simulink model "TorqueVectoring"  (R2021b)
settings: Solver=FixedStepDiscrete  StartTime=0.0  StopTime=10.0  FixedStep=0.001  RelTol=1e-3
model workspace (MAT data in the model file):
  DeadzoneYawrateError = 10
  SteeringDeadzonelimit = 10
values from neighbouring files (symbols this model uses):
  feedforwardgain = 4    [Controllerparameters.m]
  g = 9.81    [Controllerparameters.m]
  Gr = 12    [Controllerparameters.m]
  Ku = 0    [Controllerparameters.m]
  l = 1.53    [Controllerparameters.m]
  LowerYawMoment = -3600    [Controllerparameters.m]
  myy = 2    [Controllerparameters.m]
  Rd = 0.205    [Controllerparameters.m]
  Sgr = 5    [Controllerparameters.m]
  UpperYawMoment = 3600    [Controllerparameters.m]
  wf = 0.6    [Controllerparameters.m]
  wr = 0.6    [Controllerparameters.m]
libraries: simulink x1, mpclib x1
settings Model: Creator=E101180  LastModifiedBy=eiakim
settings OptimizationCC: DefaultParameterBehavior=Inlined  UseDivisionForNetSlopeComputation=on  GainParamInheritBuiltInType=on  UseFloatMulNetSlope=on  InlineInvariantSignals=on  PassReuseOutputArgsAs=Individual arguments  ZeroExternalMemoryAtStartup=off  ZeroInternalMemoryAtStartup=off  NoFixptDivByZeroProtection=on  EfficientFloat2IntCast=on  LifeSpan=1  OptimizeBlockOrder=speed  DifferentSizesBufferReuse=on  EfficientTunableParamExpr=on
settings DebuggingCC: ParameterTunabilityLossMsg=error  UnconnectedInputMsg=none  UnconnectedOutputMsg=none  UnconnectedLineMsg=none
settings HardwareCC: ProdBitPerPointer=32  ProdBitPerSizeT=32  ProdBitPerPtrDiffT=32  ProdLargestAtomicInteger=Long  ProdLargestAtomicFloat=Double  ProdWordSize=32  ProdLongLongMode=on  ProdHWDeviceType=ARM Compatible->ARM Cortex-M
settings ModelReferenceCC: EnableRefExpFcnMdlSchedulingChecks=off
settings SFSimCC: MATLABDynamicMemAlloc=off
settings RTWCC: Description=Embedded Coder  SystemTargetFile=ert.tlc  TemplateMakefile=ert_default_tmf  DLArmComputeVersion=20.02.1
settings CodeAppCC: ForceParamTrailComments=on  IgnoreCustomStorageClasses=off  OperatorAnnotations=on  SimulinkDataObjDesc=on  SFDataObjDesc=on  CustomSymbolStrGlobalVar=rt$N$M  CustomSymbolStrType=$N$M  CustomSymbolStrFcn=$N$M$F  CustomSymbolStrMacro=$N$M  InsertBlockDesc=on
settings ERTTargetCC: TargetLangStandard=C99 (ISO)  GenerateSampleERTMain=on  IncludeMdlTerminateFcn=off  CombineSignalStateStructs=on  SupportAbsoluteTime=off  SupportComplex=off  SupportNonInlinedSFcns=on  InlinedParameterPlacement=NonHierarchical  ERTCustomFileTemplate=example_file_process.tlc  ERTFilePackagingFormat=CompactWithDataFile

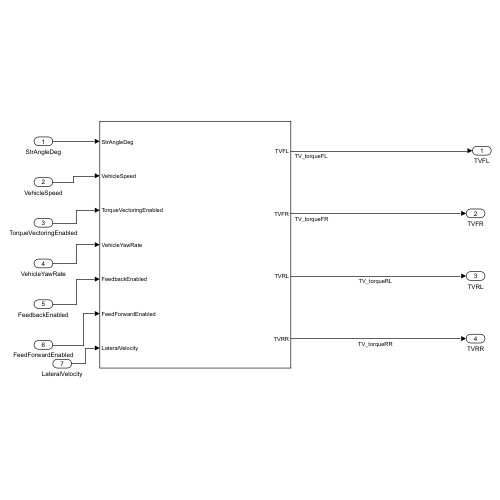
[thumbnail: Simulink's stored preview of the top-level diagram]
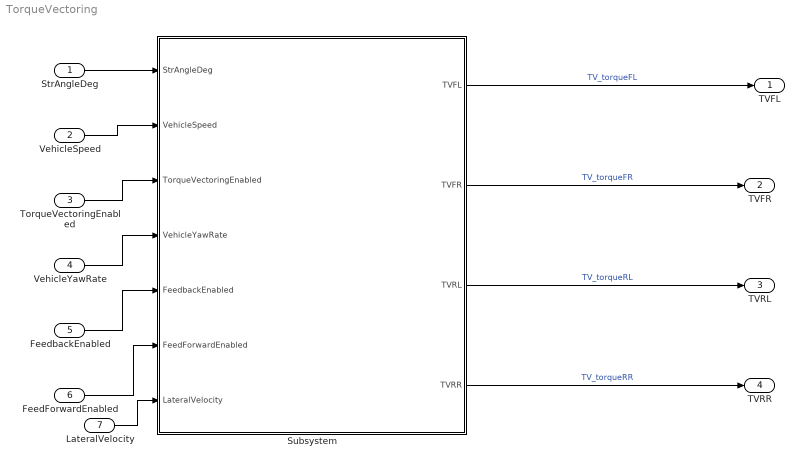
== system TorqueVectoring ==
  StrAngleDeg : Inport
  VehicleSpeed : Inport  Port=2
  TorqueVectoringEnabled : Inport  Port=3
  VehicleYawRate : Inport  Port=4
  FeedbackEnabled : Inport  Port=5
  FeedForwardEnabled : Inport  Port=6
  LateralVelocity : Inport  Port=7
  Subsystem : Subsystem
  TVFL : Outport
  TVFR : Outport  Port=2
  TVRL : Outport  Port=3
  TVRR : Outport  Port=4
  wires:
  Subsystem/3(TVRL) -> TVRL/1  "TV_torqueRL"
  Subsystem/4(TVRR) -> TVRR/1  "TV_torqueRR"
  Subsystem/1(TVFL) -> TVFL/1  "TV_torqueFL"
  StrAngleDeg/1 -> Subsystem/1(StrAngleDeg)
  VehicleSpeed/1 -> Subsystem/2(VehicleSpeed)
  TorqueVectoringEnabled/1 -> Subsystem/3(TorqueVectoringEnabled)
  FeedForwardEnabled/1 -> Subsystem/6(FeedForwardEnabled)
  FeedbackEnabled/1 -> Subsystem/5(FeedbackEnabled)
  VehicleYawRate/1 -> Subsystem/4(VehicleYawRate)
  Subsystem/2(TVFR) -> TVFR/1  "TV_torqueFR"
  LateralVelocity/1 -> Subsystem/7(LateralVelocity)

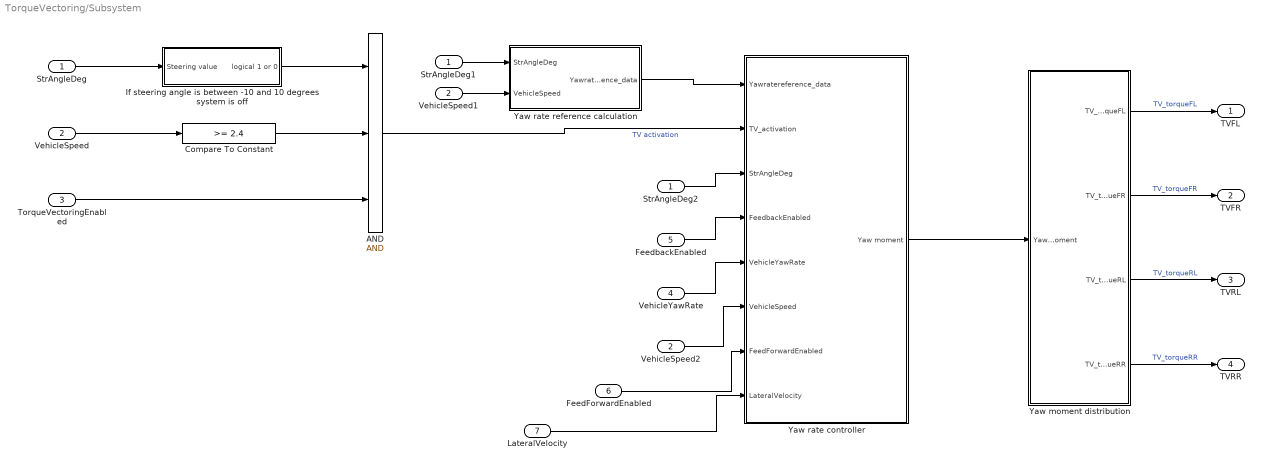
== system TorqueVectoring/Subsystem ==
  StrAngleDeg : Inport
  VehicleSpeed : Inport  Port=2
  TorqueVectoringEnabled : Inport  Port=3
  VehicleYawRate : Inport  Port=4
  FeedbackEnabled : Inport  Port=5
  FeedForwardEnabled : Inport  Port=6
  LateralVelocity : Inport  Port=7
  AND : Logic  Inputs=3  AllPortsSameDT=off  OutDataTypeStr=boolean
  Compare To Constant : simulink/Logic and Bit Operations/Compare To Constant  relop=>=  const=2.4  OutDataTypeStr=boolean
  "If steering angle is between -10 and 10 degrees system is off " : Subsystem
  StrAngleDeg1 : InportShadow
  StrAngleDeg2 : InportShadow
  VehicleSpeed1 : InportShadow  Port=2
  VehicleSpeed2 : InportShadow  Port=2
  Yaw moment distribution : Subsystem
  Yaw rate controller : Subsystem
  Yaw rate reference calculation : Subsystem
  TVFL : Outport
  TVFR : Outport  Port=2
  TVRL : Outport  Port=3
  TVRR : Outport  Port=4
  wires:
  VehicleSpeed2/1 -> Yaw rate controller/6(VehicleSpeed)
  StrAngleDeg1/1 -> Yaw rate reference calculation/1(StrAngleDeg)
  "If steering angle is between -10 and 10 degrees system is off "/1(logical 1 or 0) -> AND/1
  Yaw rate controller/1(Yaw moment) -> Yaw moment distribution/1(Yaw moment)
  VehicleSpeed/1 -> Compare To Constant/1
  StrAngleDeg/1 -> "If steering angle is between -10 and 10 degrees system is off "/1(Steering value)
  Yaw rate reference calculation/1(Yawratereference_data) -> Yaw rate controller/1(Yawratereference_data)
  AND/1 -> Yaw rate controller/2(TV_activation)  "TV activation"
  Compare To Constant/1 -> AND/2
  Yaw moment distribution/1(TV_torqueFL) -> TVFL/1  "TV_torqueFL"
  Yaw moment distribution/2(TV_torqueFR) -> TVFR/1  "TV_torqueFR"
  Yaw moment distribution/3(TV_torqueRL) -> TVRL/1  "TV_torqueRL"
  Yaw moment distribution/4(TV_torqueRR) -> TVRR/1  "TV_torqueRR"
  VehicleSpeed1/1 -> Yaw rate reference calculation/2(VehicleSpeed)
  VehicleYawRate/1 -> Yaw rate controller/5(VehicleYawRate)
  StrAngleDeg2/1 -> Yaw rate controller/3(StrAngleDeg)
  FeedbackEnabled/1 -> Yaw rate controller/4(FeedbackEnabled)
  FeedForwardEnabled/1 -> Yaw rate controller/7(FeedForwardEnabled)
  TorqueVectoringEnabled/1 -> AND/3
  LateralVelocity/1 -> Yaw rate controller/8(LateralVelocity)

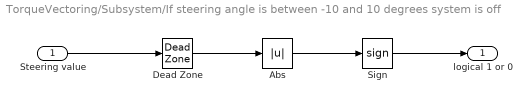
== system TorqueVectoring/Subsystem/If steering angle is between -10 and 10 degrees system is off  ==
  Steering value : Inport
  Abs : Abs
  Dead Zone : DeadZone  LowerValue=-SteeringDeadzonelimit  UpperValue=SteeringDeadzonelimit  SaturateOnIntegerOverflow=on
  Sign : Signum
  logical 1 or 0 : Outport
  wires:
  Sign/1 -> logical 1 or 0/1
  Abs/1 -> Sign/1
  Dead Zone/1 -> Abs/1
  Steering value/1 -> Dead Zone/1

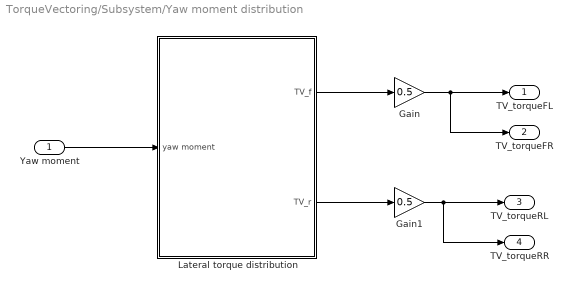
== system TorqueVectoring/Subsystem/Yaw moment distribution ==
  Yaw moment : Inport
  Gain : Gain  Gain=0.5
  Gain1 : Gain  Gain=0.5
  Lateral torque distribution : Subsystem
  TV_torqueFL : Outport
  TV_torqueFR : Outport  Port=2
  TV_torqueRL : Outport  Port=3
  TV_torqueRR : Outport  Port=4
  wires:
  Lateral torque distribution/2(TV_r) -> Gain1/1
  Lateral torque distribution/1(TV_f) -> Gain/1
  Gain/1 -> TV_torqueFL/1, TV_torqueFR/1
  Gain1/1 -> TV_torqueRR/1, TV_torqueRL/1
  Yaw moment/1 -> Lateral torque distribution/1(yaw moment)

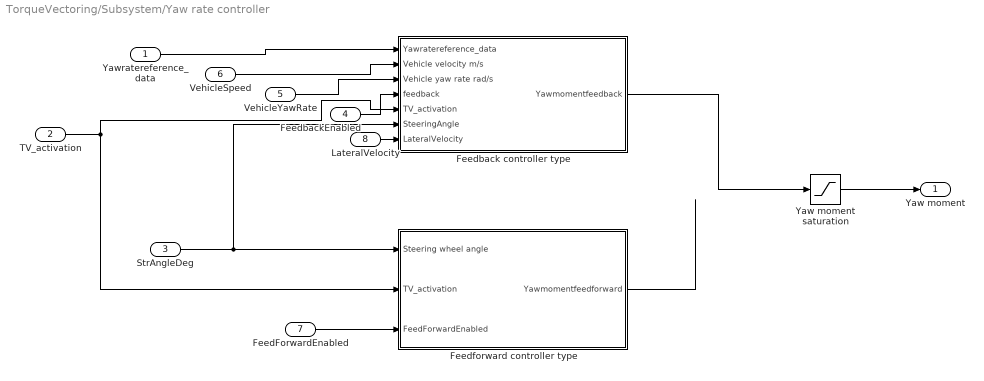
== system TorqueVectoring/Subsystem/Yaw rate controller ==
  Yawratereference_data : Inport
  TV_activation : Inport  Port=2
  StrAngleDeg : Inport  Port=3
  FeedbackEnabled : Inport  Port=4
  VehicleYawRate : Inport  Port=5
  VehicleSpeed : Inport  Port=6
  FeedForwardEnabled : Inport  Port=7
  LateralVelocity : Inport  Port=8
  Feedback controller type : Subsystem
  Feedforward controller type : Subsystem
  Yaw moment saturation : Saturate  UpperLimit=UpperYawMoment  LowerLimit=LowerYawMoment
  Yaw moment : Outport
  wires:
  Yaw moment saturation/1 -> Yaw moment/1
  FeedbackEnabled/1 -> Feedback controller type/4(feedback)
  StrAngleDeg/1 -> Feedback controller type/6(SteeringAngle), Feedforward controller type/1("Steering wheel angle ")
  VehicleYawRate/1 -> Feedback controller type/3(Vehicle yaw rate rad/s)
  VehicleSpeed/1 -> Feedback controller type/2(Vehicle velocity m/s)
  TV_activation/1 -> Feedforward controller type/2(TV_activation), Feedback controller type/5(TV_activation)
  Yawratereference_data/1 -> Feedback controller type/1(Yawratereference_data)
  Feedforward controller type/1(Yawmomentfeedforward) -> ?
  Feedback controller type/1(Yawmomentfeedback) -> Yaw moment saturation/1
  FeedForwardEnabled/1 -> Feedforward controller type/3(FeedForwardEnabled)
  LateralVelocity/1 -> Feedback controller type/7(LateralVelocity)

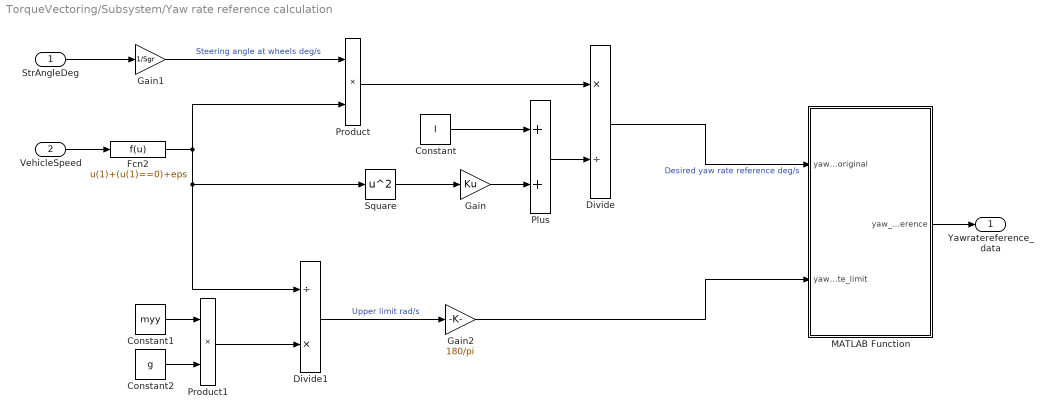
== system TorqueVectoring/Subsystem/Yaw rate reference calculation ==
  StrAngleDeg : Inport
  VehicleSpeed : Inport  Port=2
  Constant : Constant  Value=l
  Constant1 : Constant  Value=myy
  Constant2 : Constant  Value=g
  Divide : Product  Inputs=*/
  Divide1 : Product  Inputs=/*
  Fcn2 : Fcn  Expr=u(1)+(u(1)==0)+eps
  Gain : Gain  Gain=Ku
  Gain1 : Gain  Gain=1/Sgr
  Gain2 : Gain  Gain=180/pi
  MATLAB Function : MATLAB Function  TreatAsAtomicUnit=on
  Plus : Sum
  Product : Product
  Product1 : Product
  Square : Math  Operator=square  SaturateOnIntegerOverflow=on
  Yawratereference_data : Outport
  wires:
  Fcn2/1 -> Square/1, Divide1/1, Product/2
  VehicleSpeed/1 -> Fcn2/1
  Divide1/1 -> Gain2/1  "Upper limit rad/s"
  Product1/1 -> Divide1/2
  Constant2/1 -> Product1/2
  Constant1/1 -> Product1/1
  Divide/1 -> MATLAB Function/1(yaw_rate_reference_original)  "Desired yaw rate reference deg/s"
  Gain1/1 -> Product/1  "Steering angle at wheels deg/s"
  Square/1 -> Gain/1
  Gain/1 -> Plus/2
  Constant/1 -> Plus/1
  Plus/1 -> Divide/2
  StrAngleDeg/1 -> Gain1/1
  Gain2/1 -> MATLAB Function/2(yaw_rate_limit)
  MATLAB Function/1(yaw_rate_reference) -> Yawratereference_data/1
  Product/1 -> Divide/1

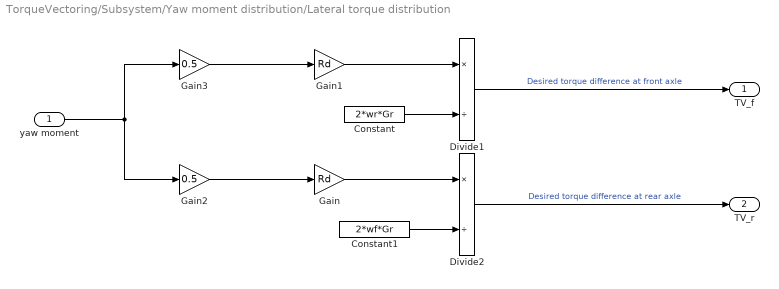
== system TorqueVectoring/Subsystem/Yaw moment distribution/Lateral torque distribution ==
  yaw moment : Inport
  Constant : Constant  Value=2*wr*Gr
  Constant1 : Constant  Value=2*wf*Gr
  Divide1 : Product  Inputs=*/
  Divide2 : Product  Inputs=*/
  Gain : Gain  Gain=Rd
  Gain1 : Gain  Gain=Rd
  Gain2 : Gain  Gain=0.5
  Gain3 : Gain  Gain=0.5
  TV_f : Outport
  TV_r : Outport  Port=2
  wires:
  yaw moment/1 -> Gain2/1, Gain3/1
  Gain3/1 -> Gain1/1
  Gain2/1 -> Gain/1
  Gain1/1 -> Divide1/1
  Gain/1 -> Divide2/1
  Divide2/1 -> TV_r/1  "Desired torque difference at rear axle"
  Divide1/1 -> TV_f/1  "Desired torque difference at front axle"
  Constant1/1 -> Divide2/2
  Constant/1 -> Divide1/2

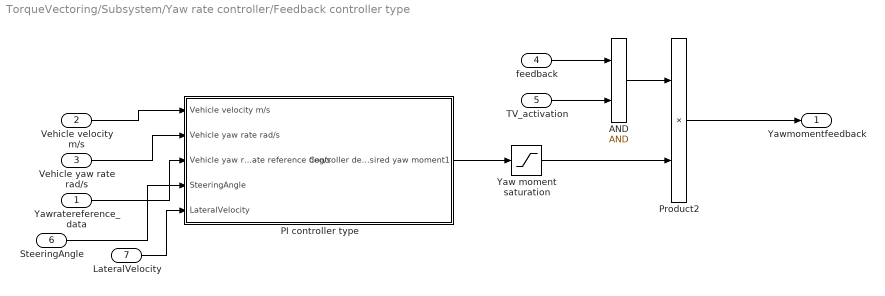
== system TorqueVectoring/Subsystem/Yaw rate controller/Feedback controller type ==
  Yawratereference_data : Inport
  Vehicle velocity m/s : Inport  Port=2
  Vehicle yaw rate rad/s : Inport  Port=3
  feedback : Inport  Port=4
  TV_activation : Inport  Port=5
  SteeringAngle : Inport  Port=6
  LateralVelocity : Inport  Port=7
  AND : Logic  AllPortsSameDT=off  OutDataTypeStr=boolean
  PI controller type : Subsystem
  Product2 : Product
  Yaw moment saturation : Saturate  UpperLimit=UpperYawMoment  LowerLimit=LowerYawMoment
  Yawmomentfeedback : Outport
  wires:
  Vehicle yaw rate rad/s/1 -> PI controller type/2(Vehicle yaw rate rad/s)
  Vehicle velocity m/s/1 -> PI controller type/1(Vehicle velocity m/s)
  feedback/1 -> AND/1
  PI controller type/1(Controller desired yaw moment1) -> Yaw moment saturation/1
  Yaw moment saturation/1 -> Product2/2
  Product2/1 -> Yawmomentfeedback/1
  AND/1 -> Product2/1
  TV_activation/1 -> AND/2
  Yawratereference_data/1 -> PI controller type/3(Vehicle yaw rate reference deg/s)
  SteeringAngle/1 -> PI controller type/4(SteeringAngle)
  LateralVelocity/1 -> PI controller type/5(LateralVelocity)

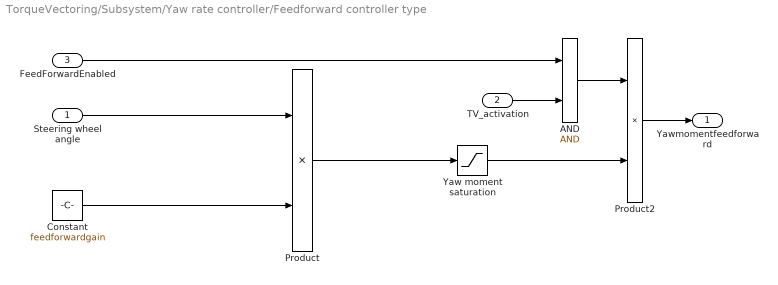
== system TorqueVectoring/Subsystem/Yaw rate controller/Feedforward controller type ==
  "Steering wheel angle " : Inport
  TV_activation : Inport  Port=2
  FeedForwardEnabled : Inport  Port=3
  AND : Logic  AllPortsSameDT=off  OutDataTypeStr=boolean
  Constant : Constant  Value=feedforwardgain
  Product : Product
  Product2 : Product
  Yaw moment saturation : Saturate  UpperLimit=UpperYawMoment  LowerLimit=LowerYawMoment
  Yawmomentfeedforward : Outport
  wires:
  "Steering wheel angle "/1 -> Product/1
  FeedForwardEnabled/1 -> AND/1
  TV_activation/1 -> AND/2
  AND/1 -> Product2/1
  Product/1 -> Yaw moment saturation/1
  Constant/1 -> Product/2
  Yaw moment saturation/1 -> Product2/2
  Product2/1 -> Yawmomentfeedforward/1

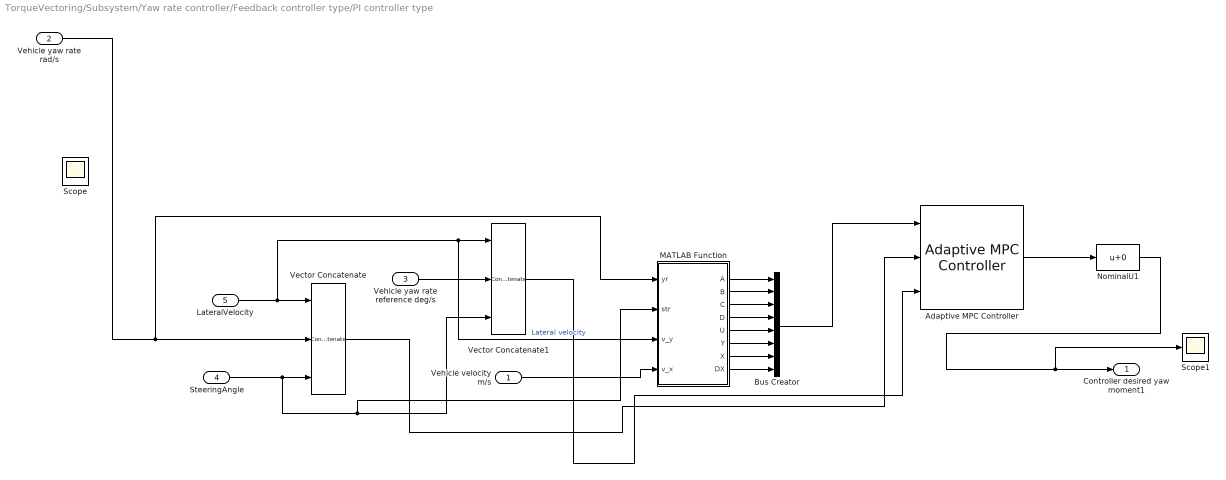
== system TorqueVectoring/Subsystem/Yaw rate controller/Feedback controller type/PI controller type ==
  Vehicle velocity m/s : Inport  PortDimensions=1
  Vehicle yaw rate rad/s : Inport  Port=2
  Vehicle yaw rate reference deg/s : Inport  Port=3
  SteeringAngle : Inport  Port=4
  LateralVelocity : Inport  Port=5
  Adaptive MPC Controller : mpclib/Adaptive MPC Controller  SCDEnableBlockLinearizationSpecification=on  mpcobj=mpc1  enable_value=0  updateMPCinCallerWorkspace=on  md_inport=off  mv_inport=off  uref_inport=off  return_cost=off  return_mvseq=off  return_qpstatus=off  return_xseq=off  return_state=off  return_ovseq=off  state_inport=off  isltv_plant=off  umin_inport=off  umax_inport=off  ymin_inport=off  ymax_inport=off  cc_inport=off  ywt_inport=off  uwt_inport=off  duwt_inport=off  rhoeps_inport=off  pm_inport=off  MaximumP=10  HorizonChoice=FixedHorizon  BlockDataType=double  SampleTimeInherited=off  switch_inport=off
  Bus Creator : BusCreator  Inputs=8
  MATLAB Function : MATLAB Function  TreatAsAtomicUnit=on
  NominalU1 : Bias  SaturateOnIntegerOverflow=on
  Scope : Scope
  Scope1 : Scope
  Vector Concatenate : Concatenate  NumInputs=3
  Vector Concatenate1 : Concatenate  NumInputs=3
  Controller desired yaw moment1 : Outport
  wires:
  Vehicle yaw rate reference deg/s/1 -> Vector Concatenate1/2
  Vehicle yaw rate rad/s/1 -> MATLAB Function/1(yr), Vector Concatenate/2
  Vector Concatenate/1 -> Adaptive MPC Controller/2
  LateralVelocity/1 -> MATLAB Function/3(v_y), Vector Concatenate1/1, Vector Concatenate/1  "Lateral velocity"
  SteeringAngle/1 -> MATLAB Function/2(str), Vector Concatenate1/3, Vector Concatenate/3
  Vector Concatenate1/1 -> Adaptive MPC Controller/3
  NominalU1/1 -> Scope1/1, Controller desired yaw moment1/1
  Adaptive MPC Controller/1 -> NominalU1/1
  MATLAB Function/1(A) -> Bus Creator/1
  MATLAB Function/2(B) -> Bus Creator/2
  MATLAB Function/3(C) -> Bus Creator/3
  MATLAB Function/4(D) -> Bus Creator/4
  MATLAB Function/5(U) -> Bus Creator/5
  MATLAB Function/6(Y) -> Bus Creator/6
  MATLAB Function/7(X) -> Bus Creator/7
  MATLAB Function/8(DX) -> Bus Creator/8
  Bus Creator/1 -> Adaptive MPC Controller/1
  Vehicle velocity m/s/1 -> MATLAB Function/4(v_x)

== matlab function TorqueVectoring/Subsystem/Yaw rate controller/Feedback controller type/PI controller type/MATLAB Function ==
  data: yr input; A output; str input; v_y input; v_x input; B output; C output; D output; U output; Y output; X output; DX output
function [A,B,C,D,U,Y,X,DX] = fcn(yr,str,v_y,v_x)

Cr = 1
Cf = 1
m = 200
Izz = 100
lf = 0.7650
lr = 0.7650


A = [-(Cr + Cf)/(m), (-v_x^2*m-Cf*lf + Cr*lr)/(m),Cf/m; (lr*Cr-lf*Cf)/(Izz), (lf^2*Cf-lr^2*Cr)/(Izz),lf*Cf/Izz;0,0,0];
B = [0; 1/Izz;0];
C = eye(3);
D = zeros([3,1]);
X = [v_y;yr;str];
Y = [v_y;yr;str];
U = [0];
%A= eye(3)+0.001*A;
%B=0.001*B;
%M=expm([A,B;zeros(1,4)]*0.001);
%A=M(1:3,1:3);
%B=M(1:3,4);
DX = A*X;

== matlab function TorqueVectoring/Subsystem/Yaw rate reference calculation/MATLAB Function ==
  data: yaw_rate_reference_original input; yaw_rate_reference output; yaw_rate_limit input
function yaw_rate_reference = fcn(yaw_rate_reference_original,yaw_rate_limit)

if abs(yaw_rate_reference_original) < yaw_rate_limit
    yaw_rate_reference = yaw_rate_reference_original ;
else 
    yaw_rate_reference = yaw_rate_limit*sign(yaw_rate_reference_original) ; 
end
